simulink library "sl_helperblocks"  (Simulink 7.5)
settings: Solver=ode45  SolverMode=SingleTasking  StartTime=0.0  StopTime=10.0  RelTol=1e-3
undefined symbols (not defined in the file or in its folder): NumDataPoints, OutputWordLength
libraries: simulink x2
Description:
  | Copyright 2004-2008 The MathWorks, Inc.
  | $Revision: 1.1.6.6 $
settings Model: Creator=andyb  LastModifiedBy=vmellark  ExtModeAutoUpdateStatusClock=off

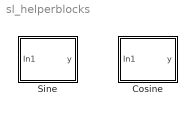
== system sl_helperblocks ==
  Cosine : Subsystem  mask(Cosine){NumDataPoints=NumDataPoints, OutputWordLength=OutputWordLength}
      mask prompts: NumDataPoints "Number of data points for lookup table:"; OutputWordLength "Output word length:"
      mask help:
      | Implement a Cosine function in Fixed-Point using a lookup table approach that exploits quarter wave symmetry.  The output fraction length equals output word length minus 2.
      |
      | The most efficient implementation is obtained when the number of data points is a power of 2 plus 1.  For example, (2^5)+1.
      mask init:
      | XData = linspace(0,0.25,NumDataPoints);
      | %
      | % using sin for the data is not a mistake.
      | % parameter pooling will cause the data for similar sines and cosines to
      | % be shared.  This can save significant amounts of ROM.
      | %
      | YData = sin(2*pi*XData);
      | OutputFracLength = OutputWordLength-2;
      | slsincoslut(gcb,XData,OutputWordLength);
      mask Display: disp('cos(2*pi*u)')
  Sine : Subsystem  mask(Sine){NumDataPoints=NumDataPoints, OutputWordLength=OutputWordLength}
      mask prompts: NumDataPoints "Number of data points for lookup table:"; OutputWordLength "Output word length:"
      mask help:
      | Implement a Sine function in Fixed-Point using a lookup table approach that exploits quarter wave symmetry.  The output fraction length equals output word length minus 2.
      |
      | The most efficient implementation is obtained when the number of data points is a power of 2 plus 1.  For example, (2^5)+1.
      mask init:
      | XData = linspace(0,0.25,NumDataPoints);
      | YData = sin(2*pi*XData);
      | OutputFracLength = OutputWordLength-2;
      | slsincoslut(gcb,XData,OutputWordLength);
      mask Display: disp('sin(2*pi*u)')

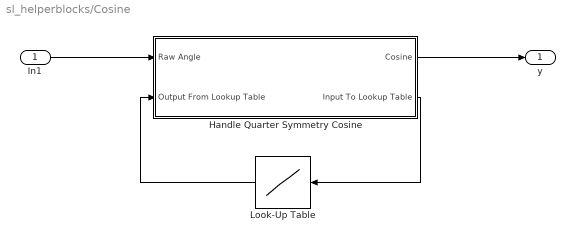
== system sl_helperblocks/Cosine ==
  In1 : Inport  OutDataType=sfix(16)  OutScaling=2^0
  Handle Quarter Symmetry Cosine : Subsystem
      mask Type: Fixed-Point-Private Quandrant Processing Sine
      mask Description:
      | This is a PRIVATE helper block not intended for direct use by customers.
      | This block manages the four possible quandrants that the input signal can be in.  Combining this block with a look up table allows the Sine function to be implemented with 75% less table data.  Only data from the first quandrant is needed.
  Look-Up Table : Lookup_n-D  NumberOfTableDimensions=1  BreakpointsForDimension1=XData  IndexSearchMethod=Evenly spaced points  Table=YData  ExtrapMethod=None - Clip  OutDataTypeStr=fixdt(1, OutputWordLength, OutputFracLength)  LockScale=on
  y : Outport  OutDataType=sfix(16)  OutScaling=2^0
  wires:
  Handle Quarter Symmetry Cosine/1(Cosine) -> y/1
  In1/1 -> Handle Quarter Symmetry Cosine/1(Raw Angle)
  Look-Up Table/1 -> Handle Quarter Symmetry Cosine/2(Output From Lookup Table)
  Handle Quarter Symmetry Cosine/2(Input To Lookup Table) -> Look-Up Table/1

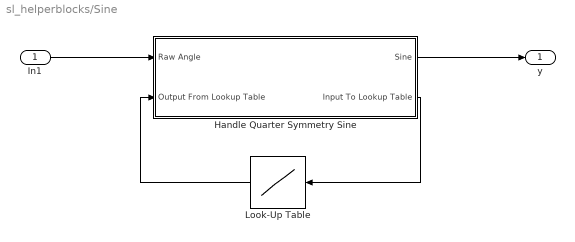
== system sl_helperblocks/Sine ==
  In1 : Inport  OutDataType=sfix(16)  OutScaling=2^0
  Handle Quarter Symmetry Sine : Subsystem
      mask Type: Fixed-Point-Private Quandrant Processing Sine
      mask Description:
      | This is a PRIVATE helper block not intended for direct use by customers.
      | This block manages the four possible quandrants that the input signal can be in.  Combining this block with a look up table allows the Sine function to be implemented with 75% less table data.  Only data from the first quandrant is needed.
  Look-Up Table : Lookup_n-D  NumberOfTableDimensions=1  BreakpointsForDimension1=XData  IndexSearchMethod=Evenly spaced points  Table=YData  ExtrapMethod=None - Clip  OutDataTypeStr=fixdt(1, OutputWordLength, OutputFracLength)  LockScale=on
  y : Outport  OutDataType=sfix(16)  OutScaling=2^0
  wires:
  Handle Quarter Symmetry Sine/2(Input To Lookup Table) -> Look-Up Table/1
  Look-Up Table/1 -> Handle Quarter Symmetry Sine/2(Output From Lookup Table)
  In1/1 -> Handle Quarter Symmetry Sine/1(Raw Angle)
  Handle Quarter Symmetry Sine/1(Sine) -> y/1

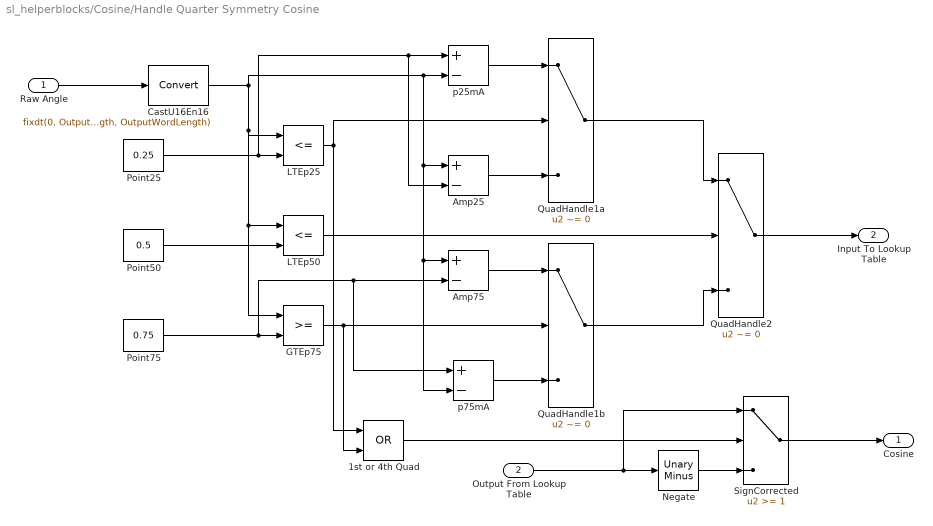
== system sl_helperblocks/Cosine/Handle Quarter Symmetry Cosine ==
  Raw Angle : Inport  OutDataType=sfix(16)  OutScaling=2^0
  Output From Lookup Table : Inport  Port=2  OutDataType=sfix(16)  OutScaling=2^0
  1st or 4th Quad : Logic  Operator=OR  AllPortsSameDT=off  OutDataTypeMode=Specify via dialog  OutDataTypeStr=uint(8)
  Amp25 : Sum  Inputs=+-  OutDataType=uint(8)  OutScaling=1  LockScale=on
  Amp75 : Sum  Inputs=+-  OutDataType=uint(8)  OutScaling=1  LockScale=on
  CastU16En16 : DataTypeConversion  OutDataTypeMode=Specify via dialog  OutDataType=fixdt(0, OutputWordLength, OutputWordLength)  OutDataTypeStr=fixdt(0, OutputWordLength, OutputWordLength)  LockScale=on
  GTEp75 : RelationalOperator  LogicOutDataTypeMode=Specify via dialog  OutDataTypeStr=uint(8)  ZeroCross=off
  LTEp25 : RelationalOperator  Operator=<=  LogicOutDataTypeMode=Specify via dialog  OutDataTypeStr=uint(8)  ZeroCross=off
  LTEp50 : RelationalOperator  Operator=<=  LogicOutDataTypeMode=Specify via dialog  OutDataTypeStr=uint(8)  ZeroCross=off
  Negate : simulink/Math Operations/Unary Minus  DoSatur=off
  Point25 : Constant  Value=0.25  OutDataTypeMode=Specify via dialog  OutDataType=fixdt(0, OutputWordLength, OutputWordLength)  ConRadixGroup=Best Precision: Vector-wise  OutDataTypeStr=fixdt(0, OutputWordLength, OutputWordLength)
  Point50 : Constant  Value=0.5  OutDataTypeMode=Specify via dialog  OutDataType=fixdt(0, OutputWordLength, OutputWordLength)  ConRadixGroup=Best Precision: Vector-wise  OutDataTypeStr=fixdt(0, OutputWordLength, OutputWordLength)
  Point75 : Constant  Value=0.75  OutDataTypeMode=Specify via dialog  OutDataType=fixdt(0, OutputWordLength, OutputWordLength)  ConRadixGroup=Best Precision: Vector-wise  OutDataTypeStr=fixdt(0, OutputWordLength, OutputWordLength)
  QuadHandle1a : Switch  Criteria=u2 ~= 0  ZeroCross=off
  QuadHandle1b : Switch  Criteria=u2 ~= 0  ZeroCross=off
  QuadHandle2 : Switch  Criteria=u2 ~= 0  ZeroCross=off
  SignCorrected : Switch  Threshold=1  ZeroCross=off
  p25mA : Sum  Inputs=+-  OutDataType=uint(8)  OutScaling=1  LockScale=on
  p75mA : Sum  Inputs=+-  OutDataType=uint(8)  OutScaling=1  LockScale=on
  Cosine : Outport  OutDataType=sfix(16)  OutScaling=2^0
  Input To Lookup Table : Outport  Port=2  OutDataType=sfix(16)  OutScaling=2^0
  wires:
  Raw Angle/1 -> CastU16En16/1
  Point25/1 -> LTEp25/2, p25mA/1, Amp25/2
  Output From Lookup Table/1 -> Negate/1, SignCorrected/1
  SignCorrected/1 -> Cosine/1
  Negate/1 -> SignCorrected/3
  CastU16En16/1 -> LTEp25/1, LTEp50/1, GTEp75/1, p25mA/2, Amp25/1, Amp75/1, p75mA/2
  Point75/1 -> GTEp75/2, Amp75/2, p75mA/1
  p25mA/1 -> QuadHandle1a/1
  Point50/1 -> LTEp50/2
  Amp25/1 -> QuadHandle1a/3
  LTEp50/1 -> QuadHandle2/2
  LTEp25/1 -> QuadHandle1a/2, 1st or 4th Quad/1
  Amp75/1 -> QuadHandle1b/1
  p75mA/1 -> QuadHandle1b/3
  GTEp75/1 -> QuadHandle1b/2, 1st or 4th Quad/2
  QuadHandle1a/1 -> QuadHandle2/1
  QuadHandle1b/1 -> QuadHandle2/3
  QuadHandle2/1 -> Input To Lookup Table/1
  1st or 4th Quad/1 -> SignCorrected/2

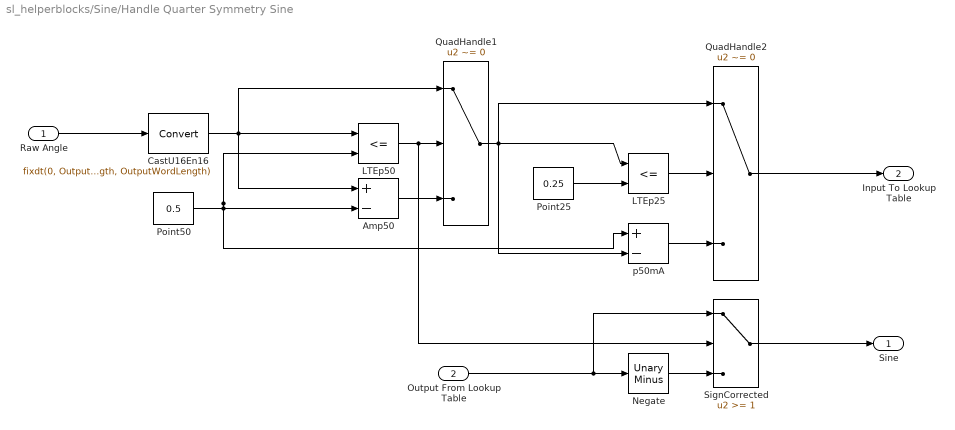
== system sl_helperblocks/Sine/Handle Quarter Symmetry Sine ==
  Raw Angle : Inport  OutDataType=sfix(16)  OutScaling=2^0
  Output From Lookup Table : Inport  Port=2  OutDataType=sfix(16)  OutScaling=2^0
  Amp50 : Sum  Inputs=+-  OutDataType=uint(8)  OutScaling=1  LockScale=on
  CastU16En16 : DataTypeConversion  OutDataTypeMode=Specify via dialog  OutDataType=fixdt(0, OutputWordLength, OutputWordLength)  OutDataTypeStr=fixdt(0, OutputWordLength, OutputWordLength)  LockScale=on
  LTEp25 : RelationalOperator  Operator=<=  LogicOutDataTypeMode=Specify via dialog  OutDataTypeStr=uint(8)  ZeroCross=off
  LTEp50 : RelationalOperator  Operator=<=  LogicOutDataTypeMode=Specify via dialog  OutDataTypeStr=uint(8)  ZeroCross=off
  Negate : simulink/Math Operations/Unary Minus  DoSatur=off
  Point25 : Constant  Value=0.25  OutDataTypeMode=Specify via dialog  OutDataType=fixdt(0, OutputWordLength, OutputWordLength)  ConRadixGroup=Best Precision: Vector-wise  OutDataTypeStr=fixdt(0, OutputWordLength, OutputWordLength)
  Point50 : Constant  Value=0.5  OutDataTypeMode=Specify via dialog  OutDataType=fixdt(0, OutputWordLength, OutputWordLength)  ConRadixGroup=Best Precision: Vector-wise  OutDataTypeStr=fixdt(0, OutputWordLength, OutputWordLength)
  QuadHandle1 : Switch  Criteria=u2 ~= 0  ZeroCross=off
  QuadHandle2 : Switch  Criteria=u2 ~= 0  ZeroCross=off
  SignCorrected : Switch  Threshold=1  ZeroCross=off
  p50mA : Sum  Inputs=+-  OutDataType=uint(8)  OutScaling=1  LockScale=on
  Sine : Outport  OutDataType=sfix(16)  OutScaling=2^0
  Input To Lookup Table : Outport  Port=2  OutDataType=sfix(16)  OutScaling=2^0
  wires:
  Point50/1 -> p50mA/1, Amp50/2, LTEp50/2
  p50mA/1 -> QuadHandle2/3
  Negate/1 -> SignCorrected/3
  Amp50/1 -> QuadHandle1/3
  SignCorrected/1 -> Sine/1
  Output From Lookup Table/1 -> SignCorrected/1, Negate/1
  CastU16En16/1 -> Amp50/1, QuadHandle1/1, LTEp50/1
  QuadHandle2/1 -> Input To Lookup Table/1
  LTEp25/1 -> QuadHandle2/2
  Point25/1 -> LTEp25/2
  QuadHandle1/1 -> p50mA/2, QuadHandle2/1, LTEp25/1
  LTEp50/1 -> SignCorrected/2, QuadHandle1/2
  Raw Angle/1 -> CastU16En16/1
